simulink model "veh_ut"  (Simulink 8.1)
settings: Solver=FixedStepDiscrete  StartTime=0.0  StopTime=10.0  FixedStep=5E-3  RelTol=1e-3
libraries: siltestlib x45, idiada_lib x11, veh x1
settings Model: Creator=xsellart  LastModifiedBy=AT015555
settings DataIOCC: SignalLoggingSaveFormat=Dataset
settings OptimizationCC: ExpressionDepthLimit=128
settings DebuggingCC: FcnCallInpInsideContextMsg=EnableAllAsError
settings GRTTargetCC: CombineOutputUpdateFcns=on  GRTInterface=off

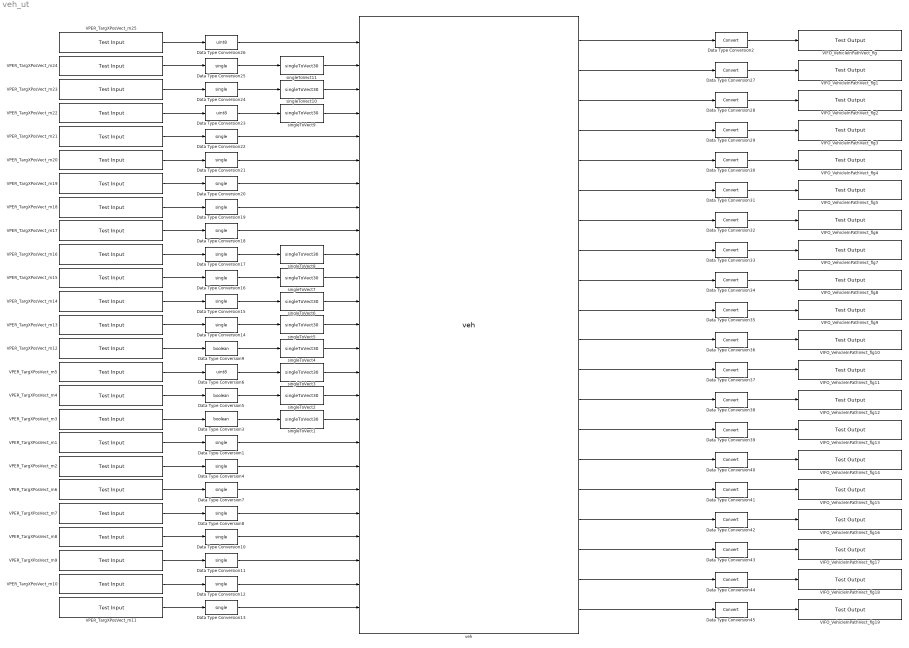
== system veh_ut ==
  Data Type Conversion{1,4,7..8,10..22,24..25} (19 alike) : DataTypeConversion  OutDataTypeStr=single
  Data Type Conversion{2,27..45} (20 alike) : DataTypeConversion
  Data Type Conversion23 : DataTypeConversion  OutDataTypeStr=uint8
  Data Type Conversion26 : DataTypeConversion  OutDataTypeStr=uint8
  Data Type Conversion3 : DataTypeConversion  OutDataTypeStr=boolean
  Data Type Conversion5 : DataTypeConversion  OutDataTypeStr=boolean
  Data Type Conversion6 : DataTypeConversion  OutDataTypeStr=uint8
  Data Type Conversion9 : DataTypeConversion  OutDataTypeStr=boolean
  VIFO_VehicleInPathVect_flg : siltestlib/Test Output  varname=VIFO_FCWMCVehId_num  sampletime=-1
  VIFO_VehicleInPathVect_flg1 : siltestlib/Test Output  varname=VIFO_AEBMCVehId_num  sampletime=-1
  VIFO_VehicleInPathVect_flg10 : siltestlib/Test Output  varname=VIFO_AEBTargetVehRelSpeedX_mps  sampletime=-1
  VIFO_VehicleInPathVect_flg11 : siltestlib/Test Output  varname=VIFO_ACCTargetVehRelSpeedX_mps  sampletime=-1
  VIFO_VehicleInPathVect_flg12 : siltestlib/Test Output  varname=VIFO_FCWMCLongAcc_mps2  sampletime=-1
  VIFO_VehicleInPathVect_flg13 : siltestlib/Test Output  varname=VIFO_AEBMCLongAcc_mps2  sampletime=-1
  VIFO_VehicleInPathVect_flg14 : siltestlib/Test Output  varname=VIFO_ACCMCLongAcc_mps2  sampletime=-1
  VIFO_VehicleInPathVect_flg15 : siltestlib/Test Output  varname=VIFO_VRUMCPedXPosition_m  sampletime=-1
  VIFO_VehicleInPathVect_flg16 : siltestlib/Test Output  varname=VIFO_VRUMCLongAcc_mps2  sampletime=-1
  VIFO_VehicleInPathVect_flg17 : siltestlib/Test Output  varname=VIFO_VRUTargetPedRelSpeedX_mps  sampletime=-1
  VIFO_VehicleInPathVect_flg18 : siltestlib/Test Output  varname=VIFO_VRUTargetPedAssigned_flg  sampletime=-1
  VIFO_VehicleInPathVect_flg19 : siltestlib/Test Output  varname=VIFO_VRUMCPedId_num  sampletime=-1
  VIFO_VehicleInPathVect_flg2 : siltestlib/Test Output  varname=VIFO_ACCMCVehId_num  sampletime=-1
  VIFO_VehicleInPathVect_flg3 : siltestlib/Test Output  varname=VIFO_FCWTargetVehAssigned_flg  sampletime=-1
  VIFO_VehicleInPathVect_flg4 : siltestlib/Test Output  varname=VIFO_AEBTargetVehAssigned_flg  sampletime=-1
  VIFO_VehicleInPathVect_flg5 : siltestlib/Test Output  varname=VIFO_ACCTargetVehAssigned_flg  sampletime=-1
  VIFO_VehicleInPathVect_flg6 : siltestlib/Test Output  varname=VIFO_FCWMCVehXPosition_m  sampletime=-1
  VIFO_VehicleInPathVect_flg7 : siltestlib/Test Output  varname=VIFO_AEBMCVehXPosition_m  sampletime=-1
  VIFO_VehicleInPathVect_flg8 : siltestlib/Test Output  varname=VIFO_ACCMCVehXPosition_m  sampletime=-1
  VIFO_VehicleInPathVect_flg9 : siltestlib/Test Output  varname=VIFO_FCWTargetVehRelSpeedX_mps  sampletime=-1
  VPER_TargXPosVect_m1 : siltestlib/Test Input  varname=VPER_LaneC0L_m  sampletime=0.005
  VPER_TargXPosVect_m10 : siltestlib/Test Input  varname=VPER_LaneC2R_rat  sampletime=0.005
  VPER_TargXPosVect_m11 : siltestlib/Test Input  varname=VPER_LaneC3R_rat  sampletime=0.005
  VPER_TargXPosVect_m12 : siltestlib/Test Input  varname=VPER_RadObjValidVect30_flg  sampletime=0.005
  VPER_TargXPosVect_m13 : siltestlib/Test Input  varname=VPER_TargAccelVect30_mps2  sampletime=0.005
  VPER_TargXPosVect_m14 : siltestlib/Test Input  varname=VPER_TargExisProbVect30_num  sampletime=0.005
  VPER_TargXPosVect_m15 : siltestlib/Test Input  varname=VPER_TargAttitudeVect30_rad  sampletime=0.005
  VPER_TargXPosVect_m16 : siltestlib/Test Input  varname=VPER_TargIdVect30_num  sampletime=0.005
  VPER_TargXPosVect_m17 : siltestlib/Test Input  varname=VDINR_SteerAngle_deg  sampletime=0.005
  VPER_TargXPosVect_m18 : siltestlib/Test Input  varname=VDINR_YawRate_degps  sampletime=0.005
  VPER_TargXPosVect_m19 : siltestlib/Test Input  varname=VDINR_VehSpd_mps  sampletime=0.005
  VPER_TargXPosVect_m2 : siltestlib/Test Input  varname=VPER_LaneC1L_rad  sampletime=0.005
  VPER_TargXPosVect_m20 : siltestlib/Test Input  varname=VPER_TargWidthVect30_m  sampletime=0.005
  VPER_TargXPosVect_m21 : siltestlib/Test Input  varname=VPER_TargAbsSpeedVect30_mps  sampletime=0.005
  VPER_TargXPosVect_m22 : siltestlib/Test Input  varname=VPER_TargTypeVect30_enum  sampletime=0.005
  VPER_TargXPosVect_m23 : siltestlib/Test Input  varname=VPER_TargYPosVect30_m  sampletime=0.005
  VPER_TargXPosVect_m24 : siltestlib/Test Input  varname=VPER_TargXPosVect30_m  sampletime=0.005
  VPER_TargXPosVect_m25 : siltestlib/Test Input  varname=VPER_NumberOfTargets_enum  sampletime=0.005
  VPER_TargXPosVect_m3 : siltestlib/Test Input  varname=VPER_CamObsStatusVect30_flg  sampletime=0.005
  VPER_TargXPosVect_m4 : siltestlib/Test Input  varname=VPER_CamObsValidVect30_flg  sampletime=0.005
  VPER_TargXPosVect_m5 : siltestlib/Test Input  varname=VPER_RadDynPropertyVect30_enum  sampletime=0.005
  VPER_TargXPosVect_m6 : siltestlib/Test Input  varname=VPER_LaneC2L_rat  sampletime=0.005
  VPER_TargXPosVect_m7 : siltestlib/Test Input  varname=VPER_LaneC3L_rat  sampletime=0.005
  VPER_TargXPosVect_m8 : siltestlib/Test Input  varname=VPER_LaneC0R_m  sampletime=0.005
  VPER_TargXPosVect_m9 : siltestlib/Test Input  varname=VPER_LaneC1R_rad  sampletime=0.005
  singleToVect{1..11} (11 alike) : idiada_lib/singleToVect30
  veh : veh/veh
  wires:
  veh/1 -> Data Type Conversion2/1
  Data Type Conversion2/1 -> VIFO_VehicleInPathVect_flg/1
  VPER_TargXPosVect_m1/1 -> Data Type Conversion1/1
  VPER_TargXPosVect_m2/1 -> Data Type Conversion4/1
  VPER_TargXPosVect_m6/1 -> Data Type Conversion7/1
  VPER_TargXPosVect_m7/1 -> Data Type Conversion8/1
  VPER_TargXPosVect_m8/1 -> Data Type Conversion10/1
  VPER_TargXPosVect_m9/1 -> Data Type Conversion11/1
  VPER_TargXPosVect_m10/1 -> Data Type Conversion12/1
  VPER_TargXPosVect_m11/1 -> Data Type Conversion13/1
  Data Type Conversion4/1 -> veh/19
  Data Type Conversion13/1 -> veh/25
  Data Type Conversion1/1 -> veh/18
  Data Type Conversion8/1 -> veh/21
  Data Type Conversion7/1 -> veh/20
  Data Type Conversion12/1 -> veh/24
  Data Type Conversion11/1 -> veh/23
  Data Type Conversion10/1 -> veh/22
  VPER_TargXPosVect_m3/1 -> Data Type Conversion3/1
  Data Type Conversion3/1 -> singleToVect1/1
  singleToVect1/1 -> veh/17
  VPER_TargXPosVect_m4/1 -> Data Type Conversion5/1
  Data Type Conversion5/1 -> singleToVect2/1
  VPER_TargXPosVect_m5/1 -> Data Type Conversion6/1
  Data Type Conversion6/1 -> singleToVect3/1
  singleToVect3/1 -> veh/15
  singleToVect2/1 -> veh/16
  VPER_TargXPosVect_m12/1 -> Data Type Conversion9/1
  Data Type Conversion9/1 -> singleToVect4/1
  singleToVect4/1 -> veh/14
  VPER_TargXPosVect_m13/1 -> Data Type Conversion14/1
  Data Type Conversion14/1 -> singleToVect5/1
  singleToVect5/1 -> veh/13
  VPER_TargXPosVect_m14/1 -> Data Type Conversion15/1
  Data Type Conversion15/1 -> singleToVect6/1
  singleToVect6/1 -> veh/12
  VPER_TargXPosVect_m15/1 -> Data Type Conversion16/1
  Data Type Conversion16/1 -> singleToVect7/1
  VPER_TargXPosVect_m16/1 -> Data Type Conversion17/1
  Data Type Conversion17/1 -> singleToVect8/1
  singleToVect8/1 -> veh/10
  singleToVect7/1 -> veh/11
  VPER_TargXPosVect_m17/1 -> Data Type Conversion18/1
  Data Type Conversion18/1 -> veh/9
  VPER_TargXPosVect_m18/1 -> Data Type Conversion19/1
  Data Type Conversion19/1 -> veh/8
  VPER_TargXPosVect_m19/1 -> Data Type Conversion20/1
  Data Type Conversion20/1 -> veh/7
  VPER_TargXPosVect_m20/1 -> Data Type Conversion21/1
  Data Type Conversion21/1 -> veh/6
  VPER_TargXPosVect_m21/1 -> Data Type Conversion22/1
  Data Type Conversion22/1 -> veh/5
  VPER_TargXPosVect_m22/1 -> Data Type Conversion23/1
  Data Type Conversion23/1 -> singleToVect9/1
  singleToVect9/1 -> veh/4
  VPER_TargXPosVect_m23/1 -> Data Type Conversion24/1
  Data Type Conversion24/1 -> singleToVect10/1
  singleToVect10/1 -> veh/3
  VPER_TargXPosVect_m24/1 -> Data Type Conversion25/1
  Data Type Conversion25/1 -> singleToVect11/1
  singleToVect11/1 -> veh/2
  VPER_TargXPosVect_m25/1 -> Data Type Conversion26/1
  Data Type Conversion26/1 -> veh/1
  Data Type Conversion27/1 -> VIFO_VehicleInPathVect_flg1/1
  Data Type Conversion28/1 -> VIFO_VehicleInPathVect_flg2/1
  Data Type Conversion29/1 -> VIFO_VehicleInPathVect_flg3/1
  veh/2 -> Data Type Conversion27/1
  veh/3 -> Data Type Conversion28/1
  veh/4 -> Data Type Conversion29/1
  Data Type Conversion30/1 -> VIFO_VehicleInPathVect_flg4/1
  veh/5 -> Data Type Conversion30/1
  Data Type Conversion31/1 -> VIFO_VehicleInPathVect_flg5/1
  veh/6 -> Data Type Conversion31/1
  Data Type Conversion32/1 -> VIFO_VehicleInPathVect_flg6/1
  veh/7 -> Data Type Conversion32/1
  Data Type Conversion33/1 -> VIFO_VehicleInPathVect_flg7/1
  veh/8 -> Data Type Conversion33/1
  Data Type Conversion34/1 -> VIFO_VehicleInPathVect_flg8/1
  veh/9 -> Data Type Conversion34/1
  Data Type Conversion35/1 -> VIFO_VehicleInPathVect_flg9/1
  veh/10 -> Data Type Conversion35/1
  Data Type Conversion36/1 -> VIFO_VehicleInPathVect_flg10/1
  Data Type Conversion37/1 -> VIFO_VehicleInPathVect_flg11/1
  Data Type Conversion38/1 -> VIFO_VehicleInPathVect_flg12/1
  Data Type Conversion39/1 -> VIFO_VehicleInPathVect_flg13/1
  Data Type Conversion40/1 -> VIFO_VehicleInPathVect_flg14/1
  Data Type Conversion41/1 -> VIFO_VehicleInPathVect_flg15/1
  Data Type Conversion42/1 -> VIFO_VehicleInPathVect_flg16/1
  Data Type Conversion43/1 -> VIFO_VehicleInPathVect_flg17/1
  Data Type Conversion44/1 -> VIFO_VehicleInPathVect_flg18/1
  Data Type Conversion45/1 -> VIFO_VehicleInPathVect_flg19/1
  veh/11 -> Data Type Conversion36/1
  veh/12 -> Data Type Conversion37/1
  veh/13 -> Data Type Conversion38/1
  veh/14 -> Data Type Conversion39/1
  veh/15 -> Data Type Conversion40/1
  veh/16 -> Data Type Conversion41/1
  veh/17 -> Data Type Conversion42/1
  veh/18 -> Data Type Conversion43/1
  veh/19 -> Data Type Conversion44/1
  veh/20 -> Data Type Conversion45/1
